simulink model "PositionPIDcontrol"  (R2020b)
settings: Solver=ode45  StartTime=0.0  StopTime=5  RelTol=1e-3
values from neighbouring files (symbols this model uses):
  daq =     [params_inertial_case.mat]    (also in params_resonant_case.mat)
  drv =     [params_inertial_case.mat]    (also in params_resonant_case.mat)
  gbox =     [params_inertial_case.mat]    (also in params_resonant_case.mat)
  mld =     [params_inertial_case.mat]    (also in params_resonant_case.mat)
  mot =     [params_inertial_case.mat]    (also in params_resonant_case.mat)
  rads2rpm = 9.54929658551    [params_inertial_case.mat]    (also in params_resonant_case.mat)
  sens =     [params_inertial_case.mat]    (also in params_resonant_case.mat)
  tau_hat = 0.00714370660323    [params_estimated_LAB0.mat]
undefined symbols (not defined in the file or in its folder): Beq, ctrl, Jeq, k_spring, step_size
settings Model: Creator=39345  LastModifiedBy=utente
settings DataIOCC: ReturnWorkspaceOutputs=off

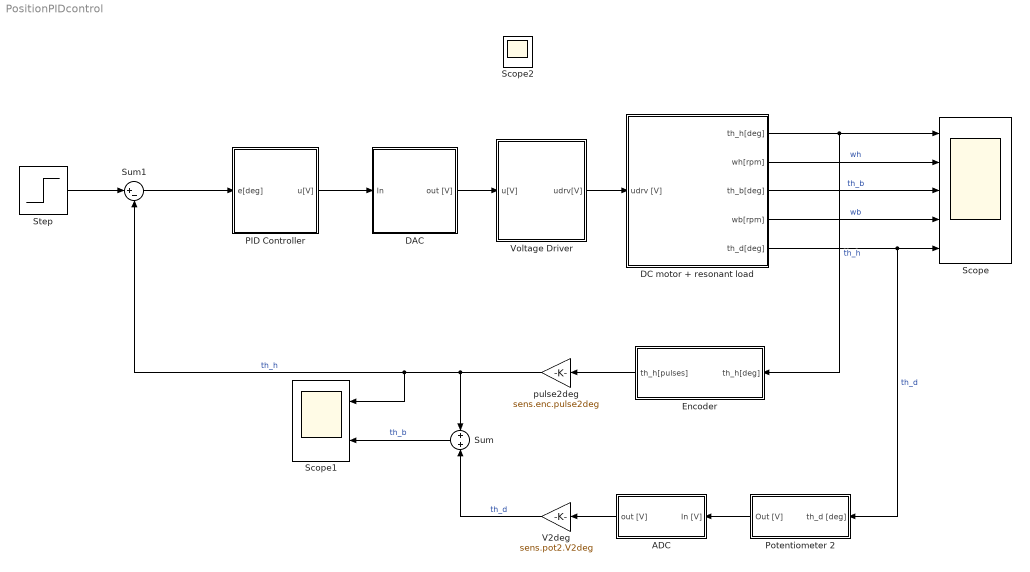
== system PositionPIDcontrol ==
  ADC : Subsystem
  DAC : Subsystem
  DC motor + resonant load : Subsystem
  Encoder : Subsystem
  PID Controller : Subsystem
  Potentiometer 2 : Subsystem
  Scope : Scope  NumInputPorts=5
  Scope1 : Scope  NumInputPorts=2
  Step : Step  After=step_size  SampleTime=0
  Sum : Sum
  Sum1 : Sum  Inputs=|+-
  V2deg : Gain  Gain=sens.pot2.V2deg
  Voltage Driver : Subsystem
  pulse2deg : Gain  Gain=sens.enc.pulse2deg
  Scope2 : Scope
  wires:
  DC motor + resonant load/1(th_h[deg]) -> Scope/1, Encoder/1(th_h[deg])  "th_h"
  DC motor + resonant load/2(wh[rpm]) -> Scope/2  "wh"
  DC motor + resonant load/4(wb[rpm]) -> Scope/4  "wb"
  DC motor + resonant load/5(th_d[deg]) -> Scope/5, Potentiometer 2/1(th_d [deg])  "th_d"
  Encoder/1(th_h[pulses]) -> pulse2deg/1
  ADC/1(out [V]) -> V2deg/1
  pulse2deg/1 -> Scope1/1, Sum1/2, Sum/1  "th_h"
  V2deg/1 -> Sum/2  "th_d"
  DAC/1(out [V]) -> Voltage Driver/1(u[V])
  Voltage Driver/1(udrv[V]) -> DC motor + resonant load/1(udrv [V])
  Potentiometer 2/1(Out [V]) -> ADC/1(In [V])
  Sum1/1 -> PID Controller/1(e[deg])
  Step/1 -> Sum1/1
  PID Controller/1(u[V]) -> DAC/1(In)
  DC motor + resonant load/3(th_b[deg]) -> Scope/3  "th_b"
  Sum/1 -> Scope1/2  "th_b"

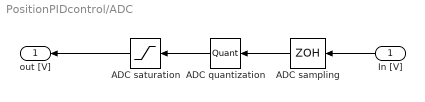
== system PositionPIDcontrol/ADC ==
  In [V] : Inport
  ADC quantization : Quantizer  QuantizationInterval=daq.dac.q
  ADC saturation : Saturate  UpperLimit=daq.dac.fs  LowerLimit=-daq.dac.fs
  ADC sampling : ZeroOrderHold  SampleTime=0.001
  out [V] : Outport
  wires:
  ADC saturation/1 -> out [V]/1
  In [V]/1 -> ADC sampling/1
  ADC quantization/1 -> ADC saturation/1
  ADC sampling/1 -> ADC quantization/1

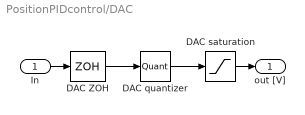
== system PositionPIDcontrol/DAC ==
  In : Inport
  DAC quantizer : Quantizer  QuantizationInterval=daq.dac.q
  DAC saturation : Saturate  UpperLimit=daq.dac.fs  LowerLimit=-daq.dac.fs
  DAC ZOH : ZeroOrderHold  SampleTime=0.001
  out [V] : Outport
  wires:
  DAC ZOH/1 -> DAC quantizer/1
  DAC quantizer/1 -> DAC saturation/1
  In/1 -> DAC ZOH/1
  DAC saturation/1 -> out [V]/1

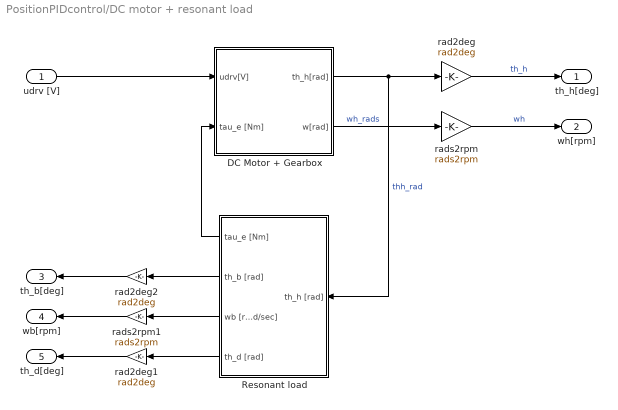
== system PositionPIDcontrol/DC motor + resonant load ==
  udrv [V] : Inport
  DC Motor + Gearbox : Subsystem
  Resonant load : Subsystem
  rad2deg : Gain  Gain=rad2deg
  rad2deg1 : Gain  Gain=rad2deg
  rad2deg2 : Gain  Gain=rad2deg
  "rads2rpm " : Gain  Gain=rads2rpm
  "rads2rpm1 " : Gain  Gain=rads2rpm
  th_h[deg] : Outport
  wh[rpm] : Outport  Port=2
  th_b[deg] : Outport  Port=3
  wb[rpm] : Outport  Port=4
  th_d[deg] : Outport  Port=5
  wires:
  Resonant load/3(wb [rad/sec]) -> "rads2rpm1 "/1
  Resonant load/4(th_d [rad]) -> rad2deg1/1
  "rads2rpm1 "/1 -> wb[rpm]/1
  rad2deg/1 -> th_h[deg]/1  "th_h"
  "rads2rpm "/1 -> wh[rpm]/1  "wh"
  rad2deg2/1 -> th_b[deg]/1
  udrv [V]/1 -> DC Motor + Gearbox/1(udrv[V])
  Resonant load/2(th_b [rad]) -> rad2deg2/1
  rad2deg1/1 -> th_d[deg]/1
  DC Motor + Gearbox/1(th_h[rad]) -> Resonant load/1(th_h [rad]), rad2deg/1  "thh_rad"
  DC Motor + Gearbox/2(w[rad]) -> "rads2rpm "/1  "wh_rads"
  Resonant load/1(tau_e [Nm]) -> DC Motor + Gearbox/2(tau_e [Nm])

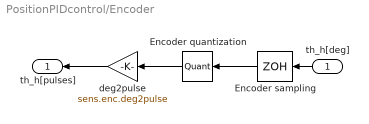
== system PositionPIDcontrol/Encoder ==
  th_h[deg] : Inport
  Encoder quantization : Quantizer  QuantizationInterval=sens.enc.pulse2deg
  Encoder sampling : ZeroOrderHold  SampleTime=-1
  deg2pulse : Gain  Gain=sens.enc.deg2pulse
  th_h[pulses] : Outport
  wires:
  th_h[deg]/1 -> Encoder sampling/1
  Encoder quantization/1 -> deg2pulse/1
  Encoder sampling/1 -> Encoder quantization/1
  deg2pulse/1 -> th_h[pulses]/1

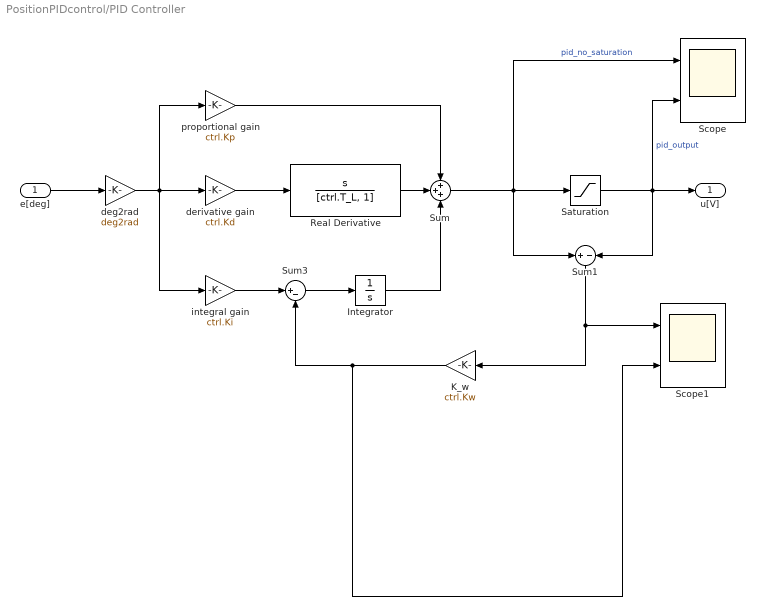
== system PositionPIDcontrol/PID Controller ==
  e[deg] : Inport
  Integrator : Integrator
  K_w : Gain  Gain=ctrl.Kw
  Real Derivative : TransferFcn  Numerator=[1 0]  Denominator=[ctrl.T_L, 1]
  Saturation : Saturate  UpperLimit=10  LowerLimit=-10
  Scope : Scope  NumInputPorts=2
  Scope1 : Scope  NumInputPorts=2
  Sum : Sum  Inputs=+++
  Sum1 : Sum  Inputs=+|-
  Sum3 : Sum  Inputs=|+-
  deg2rad : Gain  Gain=deg2rad
  derivative gain : Gain  Gain=ctrl.Kd
  integral gain : Gain  Gain=ctrl.Ki
  proportional gain : Gain  Gain=ctrl.Kp
  u[V] : Outport
  wires:
  Real Derivative/1 -> Sum/2
  proportional gain/1 -> Sum/1
  Sum1/1 -> Scope1/1, K_w/1
  derivative gain/1 -> Real Derivative/1
  deg2rad/1 -> integral gain/1, derivative gain/1, proportional gain/1
  Integrator/1 -> Sum/3
  integral gain/1 -> Sum3/1
  Sum3/1 -> Integrator/1
  K_w/1 -> Scope1/2, Sum3/2
  e[deg]/1 -> deg2rad/1
  Sum/1 -> Scope/1, Saturation/1, Sum1/1  "pid_no_saturation"
  Saturation/1 -> Scope/2, u[V]/1, Sum1/2  "pid_output"

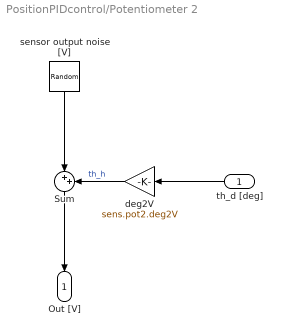
== system PositionPIDcontrol/Potentiometer 2 ==
  th_d [deg] : Inport
  Sum : Sum  Inputs=|++
  deg2V : Gain  Gain=sens.pot2.deg2V
  "sensor output noise [V] " : RandomNumber  Variance=3.5e-7  SampleTime=0.001
  Out [V] : Outport
  wires:
  th_d [deg]/1 -> deg2V/1
  deg2V/1 -> Sum/2  "th_h"
  "sensor output noise [V] "/1 -> Sum/1
  Sum/1 -> Out [V]/1

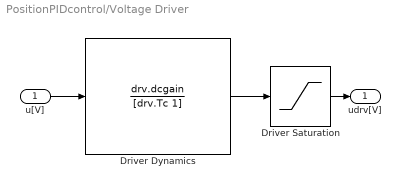
== system PositionPIDcontrol/Voltage Driver ==
  u[V] : Inport
  Driver Dynamics : TransferFcn  Numerator=drv.dcgain  Denominator=[drv.Tc 1]
  Driver Saturation : Saturate  UpperLimit=12  LowerLimit=-12
  udrv[V] : Outport
  wires:
  Driver Dynamics/1 -> Driver Saturation/1
  Driver Saturation/1 -> udrv[V]/1
  u[V]/1 -> Driver Dynamics/1

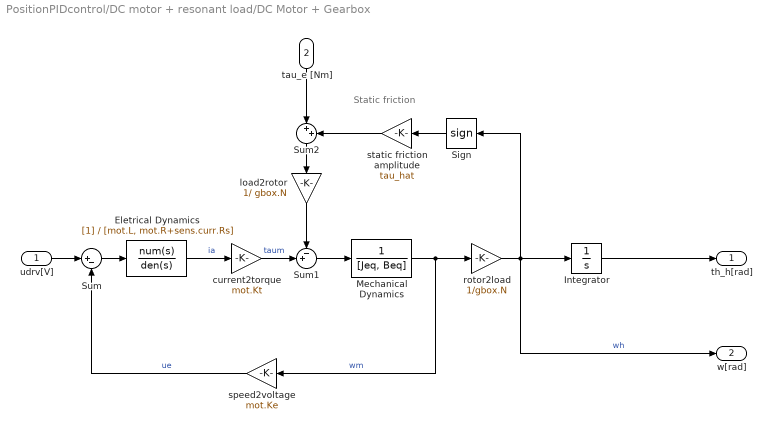
== system PositionPIDcontrol/DC motor + resonant load/DC Motor + Gearbox ==
  note: Static friction
  udrv[V] : Inport
  tau_e [Nm] : Inport  Port=2
  Eletrical Dynamics : TransferFcn  Denominator=[mot.L, mot.R+sens.curr.Rs]
  Integrator : Integrator
  Mechanical Dynamics : TransferFcn  Denominator=[Jeq, Beq]
  Sign : Signum  ZeroCross=off
  Sum : Sum  Inputs=|+-
  Sum1 : Sum  Inputs=-+|
  Sum2 : Sum  Inputs=|++
  current2torque : Gain  Gain=mot.Kt
  load2rotor : Gain  Gain=1/ gbox.N
  rotor2load : Gain  Gain=1/gbox.N
  speed2voltage : Gain  Gain=mot.Ke
  static friction amplitude : Gain  Gain=tau_hat
  th_h[rad] : Outport  VectorParamsAs1DForOutWhenUnconnected=off
  w[rad] : Outport  Port=2  VectorParamsAs1DForOutWhenUnconnected=off
  wires:
  Eletrical Dynamics/1 -> current2torque/1  "ia"
  udrv[V]/1 -> Sum/1
  Sum/1 -> Eletrical Dynamics/1
  current2torque/1 -> Sum1/2  "taum"
  Sum1/1 -> Mechanical Dynamics/1
  Mechanical Dynamics/1 -> rotor2load/1, speed2voltage/1  "wm"
  rotor2load/1 -> w[rad]/1, Integrator/1, Sign/1  "wh"
  Integrator/1 -> th_h[rad]/1
  Sign/1 -> static friction amplitude/1
  speed2voltage/1 -> Sum/2  "ue"
  load2rotor/1 -> Sum1/1
  Sum2/1 -> load2rotor/1
  static friction amplitude/1 -> Sum2/2
  tau_e [Nm]/1 -> Sum2/1

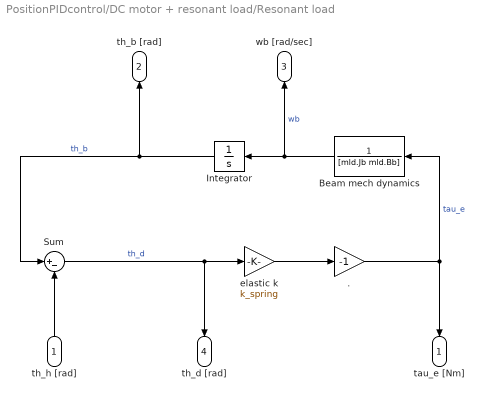
== system PositionPIDcontrol/DC motor + resonant load/Resonant load ==
  th_h [rad] : Inport
  . : Gain  Gain=-1
  Beam mech dynamics : TransferFcn  Denominator=[mld.Jb mld.Bb]
  Integrator : Integrator
  Sum : Sum  Inputs=|+-
  elastic k : Gain  Gain=k_spring
  tau_e [Nm] : Outport
  th_b [rad] : Outport  Port=2
  wb [rad/sec] : Outport  Port=3
  th_d [rad] : Outport  Port=4
  wires:
  th_h [rad]/1 -> Sum/2
  Sum/1 -> th_d [rad]/1, elastic k/1  "th_d"
  elastic k/1 -> ./1
  ./1 -> Beam mech dynamics/1, tau_e [Nm]/1  "tau_e"
  Beam mech dynamics/1 -> wb [rad/sec]/1, Integrator/1  "wb"
  Integrator/1 -> th_b [rad]/1, Sum/1  "th_b"
